simulink model "ball"  (Simulink 7.7)
settings: Solver=ode45  StartTime=0.0  StopTime=10.0  RelTol=1e-3
values from neighbouring files (symbols this model uses):
  g = 9.8000    (= 9.8)    [BEAm ball carac.m]    (also in Ball_Beam_Lead_PD.m = -9.8; bb_carac.m = -9.8)
  J = 2/5*m*R^2    (= 3.42e-06)    [BEAm ball carac.m]    (also in Ball_Beam_Lead_PD.m = 1e-06; bb_carac.m)
  m = 38*10^-3    (= 0.038)    [BEAm ball carac.m]    (also in Ball_Beam_Lead_PD.m = 0.15; bb_carac.m)
  R = 0.0150    (= 0.015)    [BEAm ball carac.m]    (also in Ball_Beam_Lead_PD.m; bb_carac.m)
settings Model: Creator=XnL  LastModifiedBy=XnL

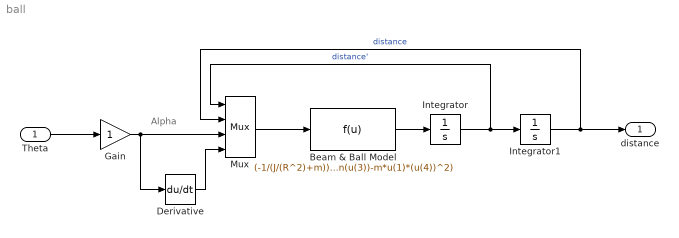
== system ball ==
  note: Alpha
  Theta : Inport
  Beam & Ball Model : Fcn  Expr=(-1/(J/(R^2)+m))*(m*g*sin(u(3))-m*u(1)*(u(4))^2)
  Derivative : Derivative
  Gain : Gain
  Integrator : Integrator
  Integrator1 : Integrator
  Mux : Mux
  distance : Outport
  wires:
  Integrator/1 -> Mux/1, Integrator1/1  "distance'"
  Integrator1/1 -> distance/1, Mux/2  "distance"
  Beam & Ball Model/1 -> Integrator/1
  Mux/1 -> Beam & Ball Model/1
  Gain/1 -> Derivative/1, Mux/3
  Derivative/1 -> Mux/4
  Theta/1 -> Gain/1
